simulink model "simulink_tutorial"  (R2018b)
settings: Solver=ode4  StartTime=0.0  StopTime=inf  FixedStep=0.05  RelTol=1e-3
undefined symbols (not defined in the file or in its folder): Angular, Linear
libraries: robotlib x3, dspstat3 x1
settings Model: Creator=ivory  LastModifiedBy=ivory
settings OptimizationCC: EnhancedBackFolding=on  PassReuseOutputArgsAs=Individual arguments  MaxStackSize=64  OptimizeBlockOrder=speed  DifferentSizesBufferReuse=on  OptimizationCustomize=off
settings DebuggingCC: ParameterTunabilityLossMsg=error
settings HardwareCC: ProdBitPerPointer=32  ProdBitPerSizeT=32  ProdBitPerPtrDiffT=32  ProdLargestAtomicFloat=None  ProdIntDivRoundTo=Undefined  ProdEndianess=Unspecified  ProdWordSize=32  ProdHWDeviceType=Generic->Unspecified (assume 32-bit Generic)
settings SFSimCC: MATLABDynamicMemAlloc=off
settings RTWCC: SystemTargetFile=ert.tlc  HardwareBoard=Robot Operating System (ROS)  TLCOptions="-aInlineSetEventsForThisBaseRateFcn=TLC_FALSE -aSuppressMultiTaskScheduler=TLC_FALSE  -aRateBasedStepFcn=0"  TemplateMakefile=ert_default_tmf  GenerateReport=on  Toolchain=Catkin  IncludeHyperlinkInReport=on  LaunchReport=on  TargetLang=C++  GenerateTraceInfo=on  GenerateTraceReport=on  GenerateTraceReportSl=on  GenerateTraceReportSf=on  GenerateTraceReportEml=on
settings CodeAppCC: ForceParamTrailComments=on  IgnoreCustomStorageClasses=off  OperatorAnnotations=on  SimulinkDataObjDesc=on  SFDataObjDesc=on  InsertBlockDesc=on
settings ERTTargetCC: SupportContinuousTime=on

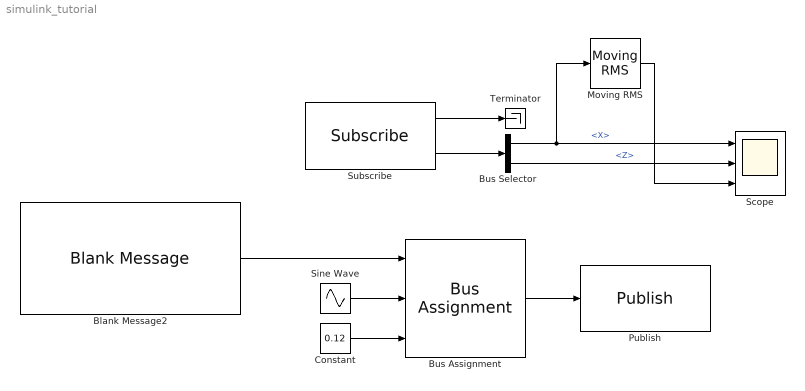
== system simulink_tutorial ==
  Blank Message2 : robotlib/Blank Message  messageClass=Message  entityType=geometry_msgs/Twist  messageType=geometry_msgs/Twist  SampleTime=inf
      settings: SourceProductBaseCode=RO
  Bus Assignment : BusAssignment  AssignedSignals=Linear.X,Angular.Z
  Bus Selector : BusSelector  OutputSignals=Linear.X,Angular.Z
  Constant : Constant  Value=0.12
  Moving RMS : dspstat3/Moving RMS  Method=Sliding window  ForgettingFactorPort=off  SpecifyWindowLength=on  WindowLength=4  ForgettingFactor=0.9  SimulateUsing=Code generation
      settings: SourceProductName=DSP System Toolbox  SourceProductBaseCode=DS
  Publish : robotlib/Publish  topicSource=Specify your own  topic=/catvehicle/cmd_vel  messageType=geometry_msgs/Twist  messageQueueLength=1
      settings: SourceProductBaseCode=RO
  Scope : Scope  NumInputPorts=3
  Sine Wave : Sin  Amplitude=4.0  Bias=4.0  SampleTime=0
  Subscribe : robotlib/Subscribe  topicSource=Specify your own  topic=/catvehicle/vel  messageType=geometry_msgs/Twist  sampleTime=-1  messageQueueLength=1
      settings: SourceProductBaseCode=RO
  Terminator : Terminator
  wires:
  Blank Message2/1 -> Bus Assignment/1
  Sine Wave/1 -> Bus Assignment/2
  Constant/1 -> Bus Assignment/3
  Bus Assignment/1 -> Publish/1
  Subscribe/1 -> Terminator/1
  Subscribe/2 -> Bus Selector/1
  Bus Selector/1 -> Moving RMS/1, Scope/1  "<X>"
  Bus Selector/2 -> Scope/2  "<Z>"
  Moving RMS/1 -> Scope/3
